simulink model "Fixed_Wing_Aircraft_Sim_ssv2"  (Simulink 10.3)
settings: Solver=VariableStepAuto  StartTime=0.0  StopTime=500  RelTol=1e-3
undefined symbols (not defined in the file or in its folder): A1_sim, A2_sim, B1_sim, B2_sim, C1_sim, C2_sim, D1_sim, D2_sim, K1_J, K1_ss, K1_u, K2_J, K2_ss, K2_u, Latr_ICs, Long_ICs
libraries: simulink_extras x8
settings Model: Creator=shahz  LastModifiedBy=shahz
settings SolverCC: AlgebraicLoopSolver=Auto
settings DataIOCC: SaveFormat=Dataset  SignalLoggingSaveFormat=Dataset  ReturnWorkspaceOutputs=on
settings OptimizationCC: ExpressionDepthLimit=128  LifeSpan=auto
settings DebuggingCC: UnderspecifiedInitializationDetection=Simplified  MergeDetectMultiDrivingBlocksExec=error  FcnCallInpInsideContextMsg=error  StateNameClashWarn=none  SFUnexpectedBacktrackingDiag=error  SFNoUnconditionalDefaultTransitionDiag=error  SFExecutionAtInitializationDiag=warning  SFMachineParentedDataDiag=error  ArithmeticOperatorsInVariantConditions=error
settings HardwareCC: ProdBitPerPointer=64  ProdBitPerSizeT=64  ProdBitPerPtrDiffT=64  ProdLargestAtomicFloat=Float  ProdIntDivRoundTo=Zero  ProdEndianess=LittleEndian  ProdWordSize=64  ProdHWDeviceType=Intel->x86-64 (Windows64)
settings ModelReferenceCC: PropagateSignalLabelsOutOfModel=on
settings SFSimCC: SimUseLocalCustomCode=on  CustomCodeUndefinedFunction=FilterOut
settings RTWCC: RTWUseLocalCustomCode=on
settings CodeAppCC: StateflowObjectComments=off
settings GRTTargetCC: TargetLangStandard=C99 (ISO)  CombineOutputUpdateFcns=on  GRTInterface=off
settings ConfigComp: CovMetricSettings=dwe  CovSaveCumulativeToWorkspaceVar=off  CovSaveSingleToWorkspaceVar=off  CovExternalEMLEnable=on

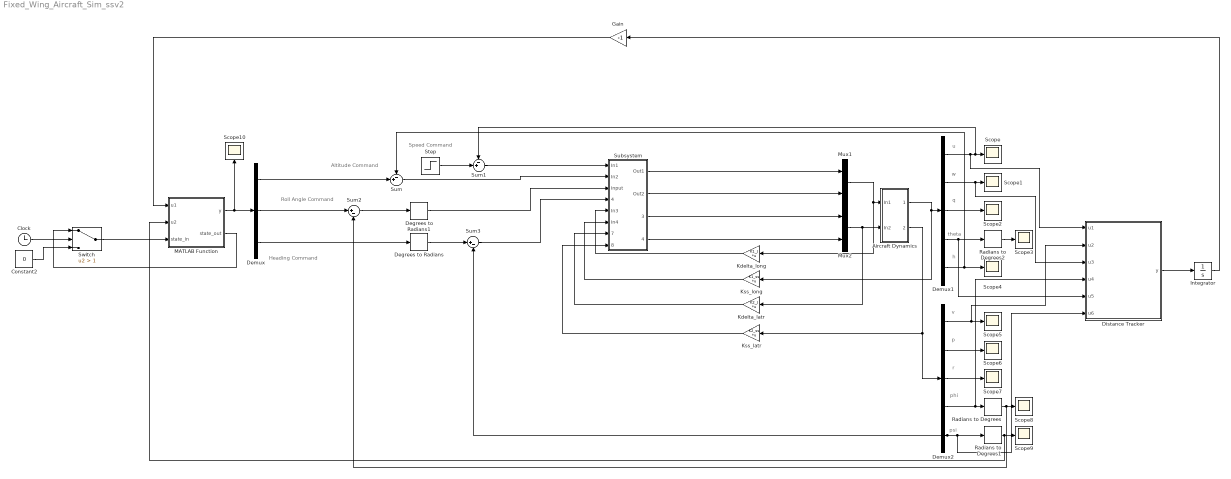
== system Fixed_Wing_Aircraft_Sim_ssv2 ==
  note: Heading Command
  note: Roll Angle Command
  note: Altitude Command
  note: Speed Command
  note: u
  note: w
  note: q
  note: theta
  note: h
  note: v
  note: p
  note: r
  note: phi
  note: psi
  Aircraft Dynamics : Subsystem
  Clock : Clock
  Constant2 : Constant  Value=0
  Degrees to Radians : simulink_extras/Transformations/Degrees to Radians
  Degrees to Radians1 : simulink_extras/Transformations/Degrees to Radians
  Demux : Demux  Outputs=3
  Demux1 : Demux  Outputs=5
  Demux2 : Demux  Outputs=5
  Distance Tracker : MATLAB Function  TreatAsAtomicUnit=on
  Gain : Gain  Gain=-1
  Integrator : Integrator
  Kdelta_latr : Gain  Gain=K2_J  Multiplication=Matrix(K*u)
  Kdelta_long : Gain  Gain=K1_J  Multiplication=Matrix(K*u)
  Kss_latr : Gain  Gain=K2_ss  Multiplication=Matrix(K*u)
  Kss_long : Gain  Gain=K1_ss  Multiplication=Matrix(K*u)
  MATLAB Function : MATLAB Function  TreatAsAtomicUnit=on
  Mux1 : Mux  Inputs=2
  Mux2 : Mux  Inputs=2
  Radians to Degrees : simulink_extras/Transformations/Radians to Degrees
  Radians to Degrees1 : simulink_extras/Transformations/Radians to Degrees
  Radians to Degrees2 : simulink_extras/Transformations/Radians to Degrees
  Scope{,1..10} (11 alike) : Scope
  Step : Step  Time=0  After=20  SampleTime=0
  Subsystem : Subsystem
  Sum : Sum  Inputs=-+|
  Sum1 : Sum  Inputs=-+|
  Sum2 : Sum  Inputs=|+-
  Sum3 : Sum  Inputs=|+-
  Switch : Switch  Criteria=u2 > Threshold  Threshold=1
  wires:
  Step/1 -> Sum1/2
  Demux1/3 -> Scope2/1
  Demux1/2 -> Distance Tracker/3(u3), Scope1/1
  Demux1/4 -> Distance Tracker/5(u5), Radians to Degrees2/1
  Demux1/5 -> Scope4/1, Sum/1
  Sum1/1 -> Subsystem/1(In1)
  Sum/1 -> Subsystem/2(In2)
  Kdelta_long/1 -> Subsystem/5(In3)
  Kss_long/1 -> Subsystem/6(In4)
  Subsystem/1(Out1) -> Mux1/1
  Subsystem/2(Out2) -> Mux1/2
  Demux2/1 -> Distance Tracker/2(u2), Scope5/1
  Demux2/5 -> Distance Tracker/6(u6), Radians to Degrees1/1, Sum3/2
  Demux2/4 -> Distance Tracker/4(u4), Radians to Degrees/1
  Demux2/2 -> Scope6/1
  Demux2/3 -> Scope7/1
  Subsystem/3(Output) -> Mux2/1
  Subsystem/4(Output1) -> Mux2/2
  Aircraft Dynamics/1(Out1) -> Kss_long/1, Demux1/1
  Mux2/1 -> Kdelta_latr/1, Aircraft Dynamics/2(In2)
  Aircraft Dynamics/2(Out2) -> Kss_latr/1, Demux2/1
  Sum2/1 -> Degrees to Radians1/1
  Sum3/1 -> Subsystem/4(Input1)
  Mux1/1 -> Kdelta_long/1, Aircraft Dynamics/1(In1)
  Degrees to Radians/1 -> Sum3/1
  Radians to Degrees/1 -> Sum2/2, Scope8/1
  Kdelta_latr/1 -> Subsystem/7(Input3)
  Kss_latr/1 -> Subsystem/8(Input2)
  Radians to Degrees2/1 -> Scope3/1
  Distance Tracker/1(y) -> Integrator/1
  Integrator/1 -> Gain/1
  Degrees to Radians1/1 -> Subsystem/3(Input)
  Demux1/1 -> Distance Tracker/1(u1), Scope/1, Sum1/1
  MATLAB Function/1(y) -> Demux/1, Scope10/1
  Demux/1 -> Sum/2
  Demux/3 -> Degrees to Radians/1
  Radians to Degrees1/1 -> MATLAB Function/2(u2), Scope9/1
  Gain/1 -> MATLAB Function/1(u1)
  Clock/1 -> Switch/2
  Switch/1 -> MATLAB Function/3(state_in)
  Constant2/1 -> Switch/3
  MATLAB Function/2(state_out) -> Switch/1
  Demux/2 -> Sum2/1

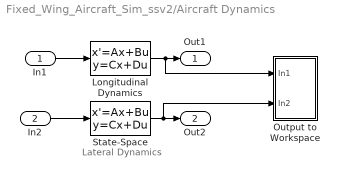
== system Fixed_Wing_Aircraft_Sim_ssv2/Aircraft Dynamics ==
  note: Lateral Dynamics
  In1 : Inport
  In2 : Inport  Port=2
  Longitudinal Dynamics : StateSpace  A=A1_sim  B=B1_sim  C=C1_sim  D=D1_sim  InitialCondition=Long_ICs  ParameterTunability=Unconstrained
  Output to Workspace : Subsystem
  State-Space : StateSpace  A=A2_sim  B=B2_sim  C=C2_sim  D=D2_sim  InitialCondition=Latr_ICs
  Out1 : Outport
  Out2 : Outport  Port=2
  wires:
  In1/1 -> Longitudinal Dynamics/1
  State-Space/1 -> Output to Workspace/2(In2), Out2/1
  In2/1 -> State-Space/1
  Longitudinal Dynamics/1 -> Output to Workspace/1(In1), Out1/1

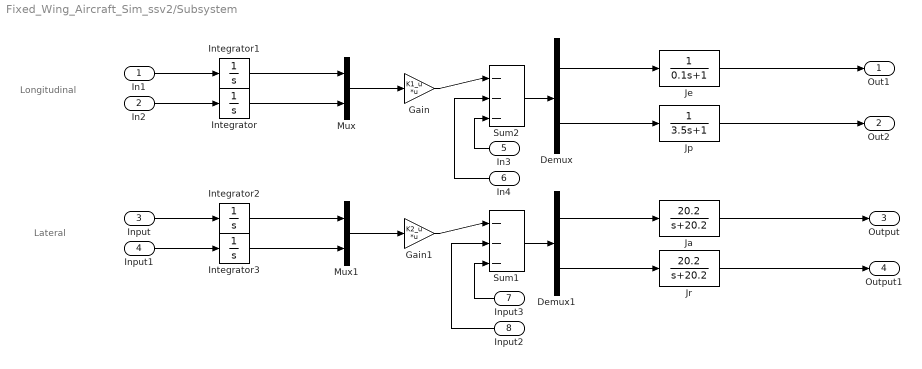
== system Fixed_Wing_Aircraft_Sim_ssv2/Subsystem ==
  note: Lateral
  note: Longitudinal
  In1 : Inport
  In2 : Inport  Port=2
  Input : Inport  Port=3
  Input1 : Inport  Port=4
  In3 : Inport  Port=5
  In4 : Inport  Port=6
  Input3 : Inport  Port=7
  Input2 : Inport  Port=8
  Demux : Demux  Outputs=2
  Demux1 : Demux  Outputs=2
  Gain : Gain  Gain=K1_u  Multiplication=Matrix(K*u)
  Gain1 : Gain  Gain=K2_u  Multiplication=Matrix(K*u)
  Integrator{,1..3} (4 alike) : Integrator
  Ja : TransferFcn  Numerator=[20.2]  Denominator=[1 20.2]
  Je : TransferFcn  Denominator="[0.1  1]"
  Jp : TransferFcn  Denominator=[3.5 1]
  Jr : TransferFcn  Numerator=[20.2]  Denominator=[1 20.2]
  Mux : Mux  Inputs=2
  Mux1 : Mux  Inputs=2
  Sum1 : Sum  Inputs=|---
  Sum2 : Sum  Inputs=|---
  Out1 : Outport
  Out2 : Outport  Port=2
  Output : Outport  Port=3
  Output1 : Outport  Port=4
  wires:
  Demux/1 -> Je/1
  Mux/1 -> Gain/1
  Sum2/1 -> Demux/1
  Demux/2 -> Jp/1
  In1/1 -> Integrator1/1
  Gain/1 -> Sum2/1
  In2/1 -> Integrator/1
  Je/1 -> Out1/1
  In4/1 -> Sum2/2
  In3/1 -> Sum2/3
  Input/1 -> Integrator2/1
  Input1/1 -> Integrator3/1
  Integrator2/1 -> Mux1/1
  Integrator3/1 -> Mux1/2
  Mux1/1 -> Gain1/1
  Gain1/1 -> Sum1/1
  Input2/1 -> Sum1/2
  Input3/1 -> Sum1/3
  Sum1/1 -> Demux1/1
  Demux1/1 -> Ja/1
  Demux1/2 -> Jr/1
  Integrator1/1 -> Mux/1
  Integrator/1 -> Mux/2
  Jp/1 -> Out2/1
  Ja/1 -> Output/1
  Jr/1 -> Output1/1

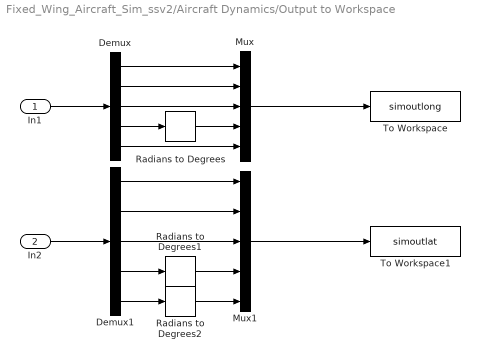
== system Fixed_Wing_Aircraft_Sim_ssv2/Aircraft Dynamics/Output to Workspace ==
  In1 : Inport
  In2 : Inport  Port=2
  Demux : Demux  Outputs=5
  Demux1 : Demux  Outputs=5
  Mux : Mux  Inputs=5
  Mux1 : Mux  Inputs=5
  Radians to Degrees : simulink_extras/Transformations/Radians to Degrees
  Radians to Degrees1 : simulink_extras/Transformations/Radians to Degrees
  Radians to Degrees2 : simulink_extras/Transformations/Radians to Degrees
  To Workspace : ToWorkspace  VariableName=simoutlong  SaveFormat=Timeseries  SampleTime=-1
  To Workspace1 : ToWorkspace  VariableName=simoutlat  SaveFormat=Timeseries  SampleTime=-1
  wires:
  In1/1 -> Demux/1
  Demux/4 -> Radians to Degrees/1
  Radians to Degrees/1 -> Mux/4
  Demux/3 -> Mux/3
  Demux/2 -> Mux/2
  Demux/1 -> Mux/1
  Demux/5 -> Mux/5
  Mux/1 -> To Workspace/1
  Mux1/1 -> To Workspace1/1
  Demux1/1 -> Mux1/1
  Demux1/2 -> Mux1/2
  Demux1/3 -> Mux1/3
  Radians to Degrees1/1 -> Mux1/4
  Demux1/4 -> Radians to Degrees1/1
  Demux1/5 -> Radians to Degrees2/1
  Radians to Degrees2/1 -> Mux1/5
  In2/1 -> Demux1/1

== matlab function Distance Tracker ==
  data: u1 input double; y output double; u2 input double; u3 input double; u4 input double; u5 input double; u6 input double
function y = fcn(u1,u2,u3,u4,u5,u6)

% u1 = u
% u2 = v
% u3 = w
% u4 = phi
% u5 = theta
% u6 = psi

y = (cos(u5)*cos(u6))*u1 + (sin(u4)*sin(u5)*cos(u6)-cos(u4)*sin(u6))*u2 + (cos(u4)*sin(u5)*cos(u6)+sin(u4)*sin(u6))*u3;

% changed the second last sin from u5 ot u4

== matlab function MATLAB Function ==
  data: u1 input double; y output double; u2 input double; state_in input double; state_out output double
function [y,state_out] = fcn(u1,u2,state_in)

% u1 is altitude and u2 is psi
if state_in <= 0
    
    state_out = 1;
    y=[2000; 0; 0];
    
else
    
    if u1<1000 && state_in < 1.5
        
        y=[2000; 0; 0];
        state_out = 1;
        
    elseif u2<180 && state_in < 2.5
        
        y=[2000; 9.26; 180];
        state_out = 2;
        
    else
        y=[1000; 0; 180];
         state_out = 3;
        
    end

end
end
